simulink subsystem "Modulador_Torque_Equivalente"  (R2026a)
settings: Solver=VariableStepAuto
settings Model: Creator=admin  LastModifiedBy=admin

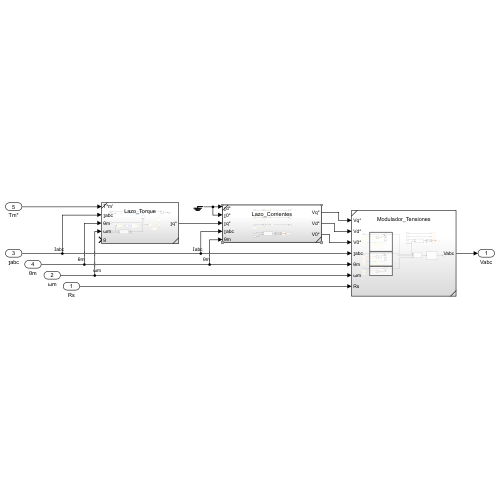
[thumbnail: Simulink's stored preview of the top-level diagram]
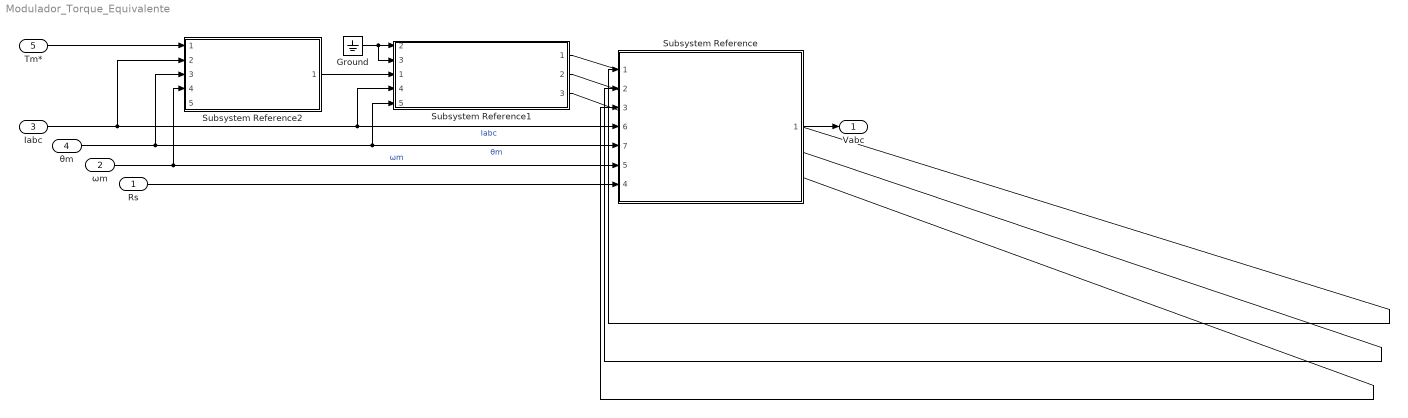
== system Modulador_Torque_Equivalente ==
  Rs : Inport
  ωm : Inport  Port=2
  Ⅰabc : Inport  Port=3
  θm : Inport  Port=4
  Tm* : Inport  Port=5
  Ground : Ground
  Subsystem Reference : Subsystem  ReferencedSubsystem=Modulador_Tensiones
      settings: PortSchema="{\"entries\":[{\"content\":{\"sides\":[{\"content\":{\"connectorIds\":[\"In1\",\"In2\",\"In3\",\"In6\",\"In7\",\"In5\",\"In4\"]},\"type\":\"ConnectorPlacement.EquallySpacedRectSide\",\"uuid\":\"561a625a-719f-47d4-85d3-a88e423068dd\"},{\"content\":{\"connectorIds\":[\"Out1\"],\"side\":\"RIGHT\"},\"type\":\"ConnectorPlacement.EquallySpacedRectSide\",\"uuid\":\"c1cdd74a-6c1d-470e-a6ac-8d72e83b5cc5\"},{\"content\":{\"side\":\"TOP\"},\"type\":\"ConnectorPlacement.EquallySpacedRectSide\",\"uuid\":\"c5935c6f-534c-46b9-aa64-6d6dabbbb210\"}]},\"type\":\"ConnectorPlacement.EquallySpacedConnector\",\"uuid\":\"b0debde9-6e18-4e06-b0c4-28c9c51e472d\"}],\"packageUris\":[\"http://schema.mathworks.com/mf0/Connector/R2020b\"],\"version\":\"1.0\"}"
  Subsystem Reference1 : Subsystem  ReferencedSubsystem=Lazo_Corrientes
      settings: PortSchema="{\"entries\":[{\"content\":{\"sides\":[{\"content\":{\"connectorIds\":[\"In2\",\"In3\",\"In1\",\"In4\",\"In5\"]},\"type\":\"ConnectorPlacement.EquallySpacedRectSide\",\"uuid\":\"7378df2b-1b9c-42cd-9ef6-9bfa4de31228\"},{\"content\":{\"connectorIds\":[\"Out1\",\"Out2\",\"Out3\"],\"side\":\"RIGHT\"},\"type\":\"ConnectorPlacement.EquallySpacedRectSide\",\"uuid\":\"75ac4e09-b611-4ee2-aa1e-16791f3f98b8\"},{\"content\":{\"side\":\"TOP\"},\"type\":\"ConnectorPlacement.EquallySpacedRectSide\",\"uuid\":\"c32b7829-5b6a-417b-8aae-eaa4caf59bef\"}]},\"type\":\"ConnectorPlacement.EquallySpacedConnector\",\"uuid\":\"1d84f5ff-db01-492a-bfe1-22065b3eebb0\"}],\"packageUris\":[\"http://schema.mathworks.com/mf0/Connector/R2020b\"],\"version\":\"1.0\"}"
  Subsystem Reference2 : Subsystem  ReferencedSubsystem=Lazo_Torque
  Vabc : Outport
  wires:
  Subsystem Reference1/1 -> Subsystem Reference/1
  Subsystem Reference1/2 -> Subsystem Reference/2
  Subsystem Reference1/3 -> Subsystem Reference/3
  Subsystem Reference2/1 -> Subsystem Reference1/1
  Tm*/1 -> Subsystem Reference2/1
  Ⅰabc/1 -> Subsystem Reference2/2, Subsystem Reference1/4, Subsystem Reference/6  "Ⅰabc"
  θm/1 -> Subsystem Reference2/3, Subsystem Reference1/5, Subsystem Reference/7  "θm"
  ωm/1 -> Subsystem Reference2/4, Subsystem Reference/5  "ωm"
  Rs/1 -> Subsystem Reference/4
  Subsystem Reference/1 -> Vabc/1
  Ground/1 -> Subsystem Reference1/3, Subsystem Reference1/2
